simulink model "gait_testing"  (R2024a)
settings: Solver=ode23t  StartTime=0.0  StopTime=8  RelTol=1e-3  AbsTol=1e-3  EnableMultiTasking=on
model workspace (MAT data in the model file):
  A = 0.4
  Length_torso : Simulink.Parameter (value not decoded)
  Lower_limbs : Simulink.Parameter (value not decoded)
  Upper_limbs : Simulink.Parameter (value not decoded)
  Width_torso : Simulink.Parameter (value not decoded)
  f = 1.5
  r_foot : Simulink.Parameter (value not decoded)
  t_leg : Simulink.Parameter (value not decoded)
symbols that are objects in the model workspace (value not decoded): Length_torso, Lower_limbs, t_leg, Upper_limbs, Width_torso
undefined symbols (not defined in the file): P0x, P0z, P1x, P1z, P2x, P2z, X, Y, Z
libraries: sm_lib x88, functionAngles x16, functionAnglesSide x16, nesl_utility x15
(part 9 of 10)

== system gait_testing/Gait Selector/Walk Left Gait - Bezier Curves/Plane Movement/Subsystem1 ==
  X(t) : Inport
  Y(t) : Inport  Port=2
  Add : Sum  Inputs=+--+
  Add1 : Sum
  Add2 : Sum
  Asin : Trigonometry  Operator=asin
  Asin1 : Trigonometry  Operator=asin
  Cos : Trigonometry  Operator=acos
  Divide : Product  Inputs=*/
  Divide1 : Product  Inputs=*/
  Gain : Gain  Gain=1/(2*Upper_limbs*Lower_limbs)
  Gain1 : Gain  Gain=Lower_limbs
  Length lower Limb : Constant  Value=Lower_limbs
  Length upper Limb : Constant  Value=Upper_limbs
  Sin : Trigonometry
  Square{,1..3} (4 alike) : Math  Operator=square
  Square Root : Sqrt
  Theta1(X,Y) : Outport
  Theta2(X,Y) : Outport  Port=2
  wires:
  X(t)/1 -> Divide/1, Square/1
  Y(t)/1 -> Square1/1
  Square/1 -> Add1/1, Add/1
  Length upper Limb/1 -> Square2/1
  Length lower Limb/1 -> Square3/1
  Square2/1 -> Add/2
  Square3/1 -> Add/3
  Square1/1 -> Add1/2, Add/4
  Add/1 -> Gain/1
  Gain/1 -> Cos/1
  Cos/1 -> Theta2(X,Y)/1, Sin/1
  Asin/1 -> Add2/1
  Sin/1 -> Gain1/1
  Add1/1 -> Square Root/1
  Gain1/1 -> Divide1/1
  Square Root/1 -> Divide/2, Divide1/2
  Divide1/1 -> Asin1/1
  Asin1/1 -> Add2/2
  Add2/1 -> Theta1(X,Y)/1
  Divide/1 -> Asin/1

== system gait_testing/Gait Selector/Walk Left Gait - Bezier Curves/Plane Movement1/Subsystem1 ==
  X(t) : Inport
  Y(t) : Inport  Port=2
  Add : Sum  Inputs=+--+
  Add1 : Sum
  Add2 : Sum
  Asin : Trigonometry  Operator=asin
  Asin1 : Trigonometry  Operator=asin
  Cos : Trigonometry  Operator=acos
  Divide : Product  Inputs=*/
  Divide1 : Product  Inputs=*/
  Gain : Gain  Gain=1/(2*Upper_limbs*Lower_limbs)
  Gain1 : Gain  Gain=Lower_limbs
  Length lower Limb : Constant  Value=Lower_limbs
  Length upper Limb : Constant  Value=Upper_limbs
  Sin : Trigonometry
  Square{,1..3} (4 alike) : Math  Operator=square
  Square Root : Sqrt
  Theta1(X,Y) : Outport
  Theta2(X,Y) : Outport  Port=2
  wires:
  X(t)/1 -> Divide/1, Square/1
  Y(t)/1 -> Square1/1
  Square/1 -> Add1/1, Add/1
  Length upper Limb/1 -> Square2/1
  Length lower Limb/1 -> Square3/1
  Square2/1 -> Add/2
  Square3/1 -> Add/3
  Square1/1 -> Add1/2, Add/4
  Add/1 -> Gain/1
  Gain/1 -> Cos/1
  Cos/1 -> Theta2(X,Y)/1, Sin/1
  Asin/1 -> Add2/1
  Sin/1 -> Gain1/1
  Add1/1 -> Square Root/1
  Gain1/1 -> Divide1/1
  Square Root/1 -> Divide/2, Divide1/2
  Divide1/1 -> Asin1/1
  Asin1/1 -> Add2/2
  Add2/1 -> Theta1(X,Y)/1
  Divide/1 -> Asin/1

== system gait_testing/Gait Selector/Walk Left Gait - Bezier Curves/Plane Movement2/Subsystem1 ==
  X(t) : Inport
  Y(t) : Inport  Port=2
  Add : Sum  Inputs=+--+
  Add1 : Sum
  Add2 : Sum
  Asin : Trigonometry  Operator=asin
  Asin1 : Trigonometry  Operator=asin
  Cos : Trigonometry  Operator=acos
  Divide : Product  Inputs=*/
  Divide1 : Product  Inputs=*/
  Gain : Gain  Gain=1/(2*Upper_limbs*Lower_limbs)
  Gain1 : Gain  Gain=Lower_limbs
  Length lower Limb : Constant  Value=Lower_limbs
  Length upper Limb : Constant  Value=Upper_limbs
  Sin : Trigonometry
  Square{,1..3} (4 alike) : Math  Operator=square
  Square Root : Sqrt
  Theta1(X,Y) : Outport
  Theta2(X,Y) : Outport  Port=2
  wires:
  Divide/1 -> Asin/1
  Add2/1 -> Theta1(X,Y)/1
  Asin1/1 -> Add2/2
  Divide1/1 -> Asin1/1
  Square Root/1 -> Divide1/2, Divide/2
  Gain1/1 -> Divide1/1
  Add1/1 -> Square Root/1
  Sin/1 -> Gain1/1
  Asin/1 -> Add2/1
  Cos/1 -> Sin/1, Theta2(X,Y)/1
  Gain/1 -> Cos/1
  Add/1 -> Gain/1
  Square1/1 -> Add/4, Add1/2
  Square3/1 -> Add/3
  Square2/1 -> Add/2
  Length lower Limb/1 -> Square3/1
  Length upper Limb/1 -> Square2/1
  Square/1 -> Add/1, Add1/1
  Y(t)/1 -> Square1/1
  X(t)/1 -> Square/1, Divide/1

== system gait_testing/Gait Selector/Walk Left Gait - Bezier Curves/Plane Movement3/Subsystem1 ==
  X(t) : Inport
  Y(t) : Inport  Port=2
  Add : Sum  Inputs=+--+
  Add1 : Sum
  Add2 : Sum
  Asin : Trigonometry  Operator=asin
  Asin1 : Trigonometry  Operator=asin
  Cos : Trigonometry  Operator=acos
  Divide : Product  Inputs=*/
  Divide1 : Product  Inputs=*/
  Gain : Gain  Gain=1/(2*Upper_limbs*Lower_limbs)
  Gain1 : Gain  Gain=Lower_limbs
  Length lower Limb : Constant  Value=Lower_limbs
  Length upper Limb : Constant  Value=Upper_limbs
  Sin : Trigonometry
  Square{,1..3} (4 alike) : Math  Operator=square
  Square Root : Sqrt
  Theta1(X,Y) : Outport
  Theta2(X,Y) : Outport  Port=2
  wires:
  X(t)/1 -> Divide/1, Square/1
  Y(t)/1 -> Square1/1
  Square/1 -> Add1/1, Add/1
  Length upper Limb/1 -> Square2/1
  Length lower Limb/1 -> Square3/1
  Square2/1 -> Add/2
  Square3/1 -> Add/3
  Square1/1 -> Add1/2, Add/4
  Add/1 -> Gain/1
  Gain/1 -> Cos/1
  Cos/1 -> Theta2(X,Y)/1, Sin/1
  Asin/1 -> Add2/1
  Sin/1 -> Gain1/1
  Add1/1 -> Square Root/1
  Gain1/1 -> Divide1/1
  Square Root/1 -> Divide/2, Divide1/2
  Divide1/1 -> Asin1/1
  Asin1/1 -> Add2/2
  Add2/1 -> Theta1(X,Y)/1
  Divide/1 -> Asin/1

== system gait_testing/Gait Selector/Walk Left Gait - Bezier Curves/Plane Movement4/Subsystem1 ==
  X(t) : Inport
  Y(t) : Inport  Port=2
  Add : Sum  Inputs=+--+
  Add1 : Sum
  Add2 : Sum
  Asin : Trigonometry  Operator=asin
  Asin1 : Trigonometry  Operator=asin
  Cos : Trigonometry  Operator=acos
  Divide : Product  Inputs=*/
  Divide1 : Product  Inputs=*/
  Gain : Gain  Gain=1/(2*Upper_limbs*Lower_limbs)
  Gain1 : Gain  Gain=Lower_limbs
  Length lower Limb : Constant  Value=Lower_limbs
  Length upper Limb : Constant  Value=Upper_limbs
  Sin : Trigonometry
  Square{,1..3} (4 alike) : Math  Operator=square
  Square Root : Sqrt
  Theta1(X,Y) : Outport
  Theta2(X,Y) : Outport  Port=2
  wires:
  Divide/1 -> Asin/1
  Add2/1 -> Theta1(X,Y)/1
  Asin1/1 -> Add2/2
  Divide1/1 -> Asin1/1
  Square Root/1 -> Divide1/2, Divide/2
  Gain1/1 -> Divide1/1
  Add1/1 -> Square Root/1
  Sin/1 -> Gain1/1
  Asin/1 -> Add2/1
  Cos/1 -> Sin/1, Theta2(X,Y)/1
  Gain/1 -> Cos/1
  Add/1 -> Gain/1
  Square1/1 -> Add/4, Add1/2
  Square3/1 -> Add/3
  Square2/1 -> Add/2
  Length lower Limb/1 -> Square3/1
  Length upper Limb/1 -> Square2/1
  Square/1 -> Add/1, Add1/1
  Y(t)/1 -> Square1/1
  X(t)/1 -> Square/1, Divide/1

== system gait_testing/Gait Selector/Walk Left Gait - Bezier Curves/Sin-Movement/Subsystem1 ==
  X(t) : Inport
  Y(t) : Inport  Port=2
  Add : Sum  Inputs=+--+
  Add1 : Sum
  Add2 : Sum
  Asin : Trigonometry  Operator=asin
  Asin1 : Trigonometry  Operator=asin
  Cos : Trigonometry  Operator=acos
  Divide : Product  Inputs=*/
  Divide1 : Product  Inputs=*/
  Gain : Gain  Gain=1/(2*Upper_limbs*Lower_limbs)
  Gain1 : Gain  Gain=Lower_limbs
  Length lower Limb : Constant  Value=Lower_limbs
  Length upper Limb : Constant  Value=Upper_limbs
  Sin : Trigonometry
  Square{,1..3} (4 alike) : Math  Operator=square
  Square Root : Sqrt
  Theta1(X,Y) : Outport
  Theta2(X,Y) : Outport  Port=2
  wires:
  X(t)/1 -> Divide/1, Square/1
  Y(t)/1 -> Square1/1
  Square/1 -> Add1/1, Add/1
  Length upper Limb/1 -> Square2/1
  Length lower Limb/1 -> Square3/1
  Square2/1 -> Add/2
  Square3/1 -> Add/3
  Square1/1 -> Add1/2, Add/4
  Add/1 -> Gain/1
  Gain/1 -> Cos/1
  Cos/1 -> Theta2(X,Y)/1, Sin/1
  Asin/1 -> Add2/1
  Sin/1 -> Gain1/1
  Add1/1 -> Square Root/1
  Gain1/1 -> Divide1/1
  Square Root/1 -> Divide/2, Divide1/2
  Divide1/1 -> Asin1/1
  Asin1/1 -> Add2/2
  Add2/1 -> Theta1(X,Y)/1
  Divide/1 -> Asin/1

== system gait_testing/Gait Selector/Walk Left Gait - Bezier Curves/Stop when change/Triggered Subsystem ==
  t : Inport
  Action Port : ActionPort  InitializeStates=reset  ActionPortLabel=case [ 1 ]:
  MATLAB Function : MATLAB Function  TreatAsAtomicUnit=on
  Change Time : Outport
  wires:
  MATLAB Function/1(activationTime) -> Change Time/1
  t/1 -> MATLAB Function/1(u)

== system gait_testing/Gait Selector/Walk Left Gait - Bezier Curves/delay and stop when change/Triggered Subsystem ==
  t : Inport
  Action Port : ActionPort  InitializeStates=reset  ActionPortLabel=case [ 1 ]:
  MATLAB Function : MATLAB Function  TreatAsAtomicUnit=on
  Change Time : Outport
  wires:
  MATLAB Function/1(activationTime) -> Change Time/1
  t/1 -> MATLAB Function/1(u)

== system gait_testing/Gait Selector/Walk Left Gait - Bezier Curves/delay and stop when change1/Triggered Subsystem ==
  t : Inport
  Action Port : ActionPort  InitializeStates=reset  ActionPortLabel=case [ 1 ]:
  MATLAB Function : MATLAB Function  TreatAsAtomicUnit=on
  Change Time : Outport
  wires:
  MATLAB Function/1(activationTime) -> Change Time/1
  t/1 -> MATLAB Function/1(u)

== system gait_testing/Gait Selector/Walk Left Gait - Bezier Curves/delay and stop when change2/Triggered Subsystem ==
  t : Inport
  Action Port : ActionPort  InitializeStates=reset  ActionPortLabel=case [ 1 ]:
  MATLAB Function : MATLAB Function  TreatAsAtomicUnit=on
  Change Time : Outport
  wires:
  MATLAB Function/1(activationTime) -> Change Time/1
  t/1 -> MATLAB Function/1(u)

== system gait_testing/Gait Selector/Walk Right Gait - Bezier Curves/Plane Movement/Subsystem1 ==
  X(t) : Inport
  Y(t) : Inport  Port=2
  Add : Sum  Inputs=+--+
  Add1 : Sum
  Add2 : Sum
  Asin : Trigonometry  Operator=asin
  Asin1 : Trigonometry  Operator=asin
  Cos : Trigonometry  Operator=acos
  Divide : Product  Inputs=*/
  Divide1 : Product  Inputs=*/
  Gain : Gain  Gain=1/(2*Upper_limbs*Lower_limbs)
  Gain1 : Gain  Gain=Lower_limbs
  Length lower Limb : Constant  Value=Lower_limbs
  Length upper Limb : Constant  Value=Upper_limbs
  Sin : Trigonometry
  Square{,1..3} (4 alike) : Math  Operator=square
  Square Root : Sqrt
  Theta1(X,Y) : Outport
  Theta2(X,Y) : Outport  Port=2
  wires:
  Divide/1 -> Asin/1
  Add2/1 -> Theta1(X,Y)/1
  Asin1/1 -> Add2/2
  Divide1/1 -> Asin1/1
  Square Root/1 -> Divide1/2, Divide/2
  Gain1/1 -> Divide1/1
  Add1/1 -> Square Root/1
  Sin/1 -> Gain1/1
  Asin/1 -> Add2/1
  Cos/1 -> Sin/1, Theta2(X,Y)/1
  Gain/1 -> Cos/1
  Add/1 -> Gain/1
  Square1/1 -> Add/4, Add1/2
  Square3/1 -> Add/3
  Square2/1 -> Add/2
  Length lower Limb/1 -> Square3/1
  Length upper Limb/1 -> Square2/1
  Square/1 -> Add/1, Add1/1
  Y(t)/1 -> Square1/1
  X(t)/1 -> Square/1, Divide/1

== system gait_testing/Gait Selector/Walk Right Gait - Bezier Curves/Plane Movement1/Subsystem1 ==
  X(t) : Inport
  Y(t) : Inport  Port=2
  Add : Sum  Inputs=+--+
  Add1 : Sum
  Add2 : Sum
  Asin : Trigonometry  Operator=asin
  Asin1 : Trigonometry  Operator=asin
  Cos : Trigonometry  Operator=acos
  Divide : Product  Inputs=*/
  Divide1 : Product  Inputs=*/
  Gain : Gain  Gain=1/(2*Upper_limbs*Lower_limbs)
  Gain1 : Gain  Gain=Lower_limbs
  Length lower Limb : Constant  Value=Lower_limbs
  Length upper Limb : Constant  Value=Upper_limbs
  Sin : Trigonometry
  Square{,1..3} (4 alike) : Math  Operator=square
  Square Root : Sqrt
  Theta1(X,Y) : Outport
  Theta2(X,Y) : Outport  Port=2
  wires:
  Divide/1 -> Asin/1
  Add2/1 -> Theta1(X,Y)/1
  Asin1/1 -> Add2/2
  Divide1/1 -> Asin1/1
  Square Root/1 -> Divide1/2, Divide/2
  Gain1/1 -> Divide1/1
  Add1/1 -> Square Root/1
  Sin/1 -> Gain1/1
  Asin/1 -> Add2/1
  Cos/1 -> Sin/1, Theta2(X,Y)/1
  Gain/1 -> Cos/1
  Add/1 -> Gain/1
  Square1/1 -> Add/4, Add1/2
  Square3/1 -> Add/3
  Square2/1 -> Add/2
  Length lower Limb/1 -> Square3/1
  Length upper Limb/1 -> Square2/1
  Square/1 -> Add/1, Add1/1
  Y(t)/1 -> Square1/1
  X(t)/1 -> Square/1, Divide/1

== system gait_testing/Gait Selector/Walk Right Gait - Bezier Curves/Plane Movement2/Subsystem1 ==
  X(t) : Inport
  Y(t) : Inport  Port=2
  Add : Sum  Inputs=+--+
  Add1 : Sum
  Add2 : Sum
  Asin : Trigonometry  Operator=asin
  Asin1 : Trigonometry  Operator=asin
  Cos : Trigonometry  Operator=acos
  Divide : Product  Inputs=*/
  Divide1 : Product  Inputs=*/
  Gain : Gain  Gain=1/(2*Upper_limbs*Lower_limbs)
  Gain1 : Gain  Gain=Lower_limbs
  Length lower Limb : Constant  Value=Lower_limbs
  Length upper Limb : Constant  Value=Upper_limbs
  Sin : Trigonometry
  Square{,1..3} (4 alike) : Math  Operator=square
  Square Root : Sqrt
  Theta1(X,Y) : Outport
  Theta2(X,Y) : Outport  Port=2
  wires:
  X(t)/1 -> Divide/1, Square/1
  Y(t)/1 -> Square1/1
  Square/1 -> Add1/1, Add/1
  Length upper Limb/1 -> Square2/1
  Length lower Limb/1 -> Square3/1
  Square2/1 -> Add/2
  Square3/1 -> Add/3
  Square1/1 -> Add1/2, Add/4
  Add/1 -> Gain/1
  Gain/1 -> Cos/1
  Cos/1 -> Theta2(X,Y)/1, Sin/1
  Asin/1 -> Add2/1
  Sin/1 -> Gain1/1
  Add1/1 -> Square Root/1
  Gain1/1 -> Divide1/1
  Square Root/1 -> Divide/2, Divide1/2
  Divide1/1 -> Asin1/1
  Asin1/1 -> Add2/2
  Add2/1 -> Theta1(X,Y)/1
  Divide/1 -> Asin/1

== system gait_testing/Gait Selector/Walk Right Gait - Bezier Curves/Plane Movement3/Subsystem1 ==
  X(t) : Inport
  Y(t) : Inport  Port=2
  Add : Sum  Inputs=+--+
  Add1 : Sum
  Add2 : Sum
  Asin : Trigonometry  Operator=asin
  Asin1 : Trigonometry  Operator=asin
  Cos : Trigonometry  Operator=acos
  Divide : Product  Inputs=*/
  Divide1 : Product  Inputs=*/
  Gain : Gain  Gain=1/(2*Upper_limbs*Lower_limbs)
  Gain1 : Gain  Gain=Lower_limbs
  Length lower Limb : Constant  Value=Lower_limbs
  Length upper Limb : Constant  Value=Upper_limbs
  Sin : Trigonometry
  Square{,1..3} (4 alike) : Math  Operator=square
  Square Root : Sqrt
  Theta1(X,Y) : Outport
  Theta2(X,Y) : Outport  Port=2
  wires:
  Divide/1 -> Asin/1
  Add2/1 -> Theta1(X,Y)/1
  Asin1/1 -> Add2/2
  Divide1/1 -> Asin1/1
  Square Root/1 -> Divide1/2, Divide/2
  Gain1/1 -> Divide1/1
  Add1/1 -> Square Root/1
  Sin/1 -> Gain1/1
  Asin/1 -> Add2/1
  Cos/1 -> Sin/1, Theta2(X,Y)/1
  Gain/1 -> Cos/1
  Add/1 -> Gain/1
  Square1/1 -> Add/4, Add1/2
  Square3/1 -> Add/3
  Square2/1 -> Add/2
  Length lower Limb/1 -> Square3/1
  Length upper Limb/1 -> Square2/1
  Square/1 -> Add/1, Add1/1
  Y(t)/1 -> Square1/1
  X(t)/1 -> Square/1, Divide/1

== system gait_testing/Gait Selector/Walk Right Gait - Bezier Curves/Plane Movement4/Subsystem1 ==
  X(t) : Inport
  Y(t) : Inport  Port=2
  Add : Sum  Inputs=+--+
  Add1 : Sum
  Add2 : Sum
  Asin : Trigonometry  Operator=asin
  Asin1 : Trigonometry  Operator=asin
  Cos : Trigonometry  Operator=acos
  Divide : Product  Inputs=*/
  Divide1 : Product  Inputs=*/
  Gain : Gain  Gain=1/(2*Upper_limbs*Lower_limbs)
  Gain1 : Gain  Gain=Lower_limbs
  Length lower Limb : Constant  Value=Lower_limbs
  Length upper Limb : Constant  Value=Upper_limbs
  Sin : Trigonometry
  Square{,1..3} (4 alike) : Math  Operator=square
  Square Root : Sqrt
  Theta1(X,Y) : Outport
  Theta2(X,Y) : Outport  Port=2
  wires:
  X(t)/1 -> Divide/1, Square/1
  Y(t)/1 -> Square1/1
  Square/1 -> Add1/1, Add/1
  Length upper Limb/1 -> Square2/1
  Length lower Limb/1 -> Square3/1
  Square2/1 -> Add/2
  Square3/1 -> Add/3
  Square1/1 -> Add1/2, Add/4
  Add/1 -> Gain/1
  Gain/1 -> Cos/1
  Cos/1 -> Theta2(X,Y)/1, Sin/1
  Asin/1 -> Add2/1
  Sin/1 -> Gain1/1
  Add1/1 -> Square Root/1
  Gain1/1 -> Divide1/1
  Square Root/1 -> Divide/2, Divide1/2
  Divide1/1 -> Asin1/1
  Asin1/1 -> Add2/2
  Add2/1 -> Theta1(X,Y)/1
  Divide/1 -> Asin/1

== system gait_testing/Gait Selector/Walk Right Gait - Bezier Curves/Sin-Movement/Subsystem1 ==
  X(t) : Inport
  Y(t) : Inport  Port=2
  Add : Sum  Inputs=+--+
  Add1 : Sum
  Add2 : Sum
  Asin : Trigonometry  Operator=asin
  Asin1 : Trigonometry  Operator=asin
  Cos : Trigonometry  Operator=acos
  Divide : Product  Inputs=*/
  Divide1 : Product  Inputs=*/
  Gain : Gain  Gain=1/(2*Upper_limbs*Lower_limbs)
  Gain1 : Gain  Gain=Lower_limbs
  Length lower Limb : Constant  Value=Lower_limbs
  Length upper Limb : Constant  Value=Upper_limbs
  Sin : Trigonometry
  Square{,1..3} (4 alike) : Math  Operator=square
  Square Root : Sqrt
  Theta1(X,Y) : Outport
  Theta2(X,Y) : Outport  Port=2
  wires:
  Divide/1 -> Asin/1
  Add2/1 -> Theta1(X,Y)/1
  Asin1/1 -> Add2/2
  Divide1/1 -> Asin1/1
  Square Root/1 -> Divide1/2, Divide/2
  Gain1/1 -> Divide1/1
  Add1/1 -> Square Root/1
  Sin/1 -> Gain1/1
  Asin/1 -> Add2/1
  Cos/1 -> Sin/1, Theta2(X,Y)/1
  Gain/1 -> Cos/1
  Add/1 -> Gain/1
  Square1/1 -> Add/4, Add1/2
  Square3/1 -> Add/3
  Square2/1 -> Add/2
  Length lower Limb/1 -> Square3/1
  Length upper Limb/1 -> Square2/1
  Square/1 -> Add/1, Add1/1
  Y(t)/1 -> Square1/1
  X(t)/1 -> Square/1, Divide/1

== system gait_testing/Gait Selector/Walk Right Gait - Bezier Curves/Stop when change/Triggered Subsystem ==
  t : Inport
  Action Port : ActionPort  InitializeStates=reset  ActionPortLabel=case [ 1 ]:
  MATLAB Function : MATLAB Function  TreatAsAtomicUnit=on
  Change Time : Outport
  wires:
  MATLAB Function/1(activationTime) -> Change Time/1
  t/1 -> MATLAB Function/1(u)

== system gait_testing/Gait Selector/Walk Right Gait - Bezier Curves/delay and stop when change/Triggered Subsystem ==
  t : Inport
  Action Port : ActionPort  InitializeStates=reset  ActionPortLabel=case [ 1 ]:
  MATLAB Function : MATLAB Function  TreatAsAtomicUnit=on
  Change Time : Outport
  wires:
  MATLAB Function/1(activationTime) -> Change Time/1
  t/1 -> MATLAB Function/1(u)

== system gait_testing/Gait Selector/Walk Right Gait - Bezier Curves/delay and stop when change1/Triggered Subsystem ==
  t : Inport
  Action Port : ActionPort  InitializeStates=reset  ActionPortLabel=case [ 1 ]:
  MATLAB Function : MATLAB Function  TreatAsAtomicUnit=on
  Change Time : Outport
  wires:
  MATLAB Function/1(activationTime) -> Change Time/1
  t/1 -> MATLAB Function/1(u)

== system gait_testing/Gait Selector/Walk Right Gait - Bezier Curves/delay and stop when change2/Triggered Subsystem ==
  t : Inport
  Action Port : ActionPort  InitializeStates=reset  ActionPortLabel=case [ 1 ]:
  MATLAB Function : MATLAB Function  TreatAsAtomicUnit=on
  Change Time : Outport
  wires:
  MATLAB Function/1(activationTime) -> Change Time/1
  t/1 -> MATLAB Function/1(u)

== matlab function gait_testing/Gait Selector/Walk Gait - Bezier Curves/delay and stop when change/Triggered Subsystem/MATLAB Function ==
  data: u input; activationTime output
function activationTime = getActivationTime(u)
    persistent t_start
    if isempty(t_start)
        t_start = u;
    end
    activationTime = t_start;
end

== matlab function gait_testing/Gait Selector/Walk Gait - Bezier Curves/delay and stop when change1/Triggered Subsystem/MATLAB Function ==
  data: u input; activationTime output
function activationTime = getActivationTime(u)
    persistent t_start
    if isempty(t_start)
        t_start = u;
    end
    activationTime = t_start;
end

== matlab function gait_testing/Gait Selector/Walk Gait - Bezier Curves/delay and stop when change2/Triggered Subsystem/MATLAB Function ==
  data: u input; activationTime output
function activationTime = getActivationTime(u)
    persistent t_start
    if isempty(t_start)
        t_start = u;
    end
    activationTime = t_start;
end

== matlab function gait_testing/Gait Selector/MATLAB Function ==
  data: c_old input; c_new input; t input; C_out output; t_change input; tdur_old input; tdur_new input; tdur_out output
function [C_out, tdur_out]= control_change(c_old, c_new, t, t_change, tdur_old, tdur_new)

time_since_change = t-t_change;
if c_old == 0 || t < tdur_old
    C_out = c_new;
    tdur_out = tdur_new;

else
    if time_since_change < tdur_old
        C_out = c_old;
        tdur_out = tdur_old;
    else
        if time_since_change < (tdur_old+0.05)
            C_out = 0;
            tdur_out = 0.05;
        else
            C_out = c_new;
            tdur_out = tdur_new;
        end
    end

end
end

== matlab function gait_testing/Gait Selector/Trot Gait - Bezier Curves/Stop when change/Triggered Subsystem/MATLAB Function ==
  data: u input; activationTime output
function activationTime = getActivationTime(u)
    persistent t_start
    if isempty(t_start)
        t_start = u;
    end
    activationTime = t_start;
end

== matlab function gait_testing/Gait Selector/Trot Gait - Bezier Curves/delay and stop when change/Triggered Subsystem/MATLAB Function ==
  data: u input; activationTime output
function activationTime = getActivationTime(u)
    persistent t_start
    if isempty(t_start)
        t_start = u;
    end
    activationTime = t_start;
end

== matlab function gait_testing/Gait Selector/Trot Gait - Bezier Curves/delay and stop when change1/Triggered Subsystem/MATLAB Function ==
  data: u input; activationTime output
function activationTime = getActivationTime(u)
    persistent t_start
    if isempty(t_start)
        t_start = u;
    end
    activationTime = t_start;
end

== matlab function gait_testing/Gait Selector/Trot Gait - Bezier Curves/delay and stop when change2/Triggered Subsystem/MATLAB Function ==
  data: u input; activationTime output
function activationTime = getActivationTime(u)
    persistent t_start
    if isempty(t_start)
        t_start = u;
    end
    activationTime = t_start;
end

== matlab function gait_testing/Gait Selector/Walk Back Gait - Bezier Curves/Stop when change/Triggered Subsystem/MATLAB Function ==
  data: u input; activationTime output
function activationTime = getActivationTime(u)
    persistent t_start
    if isempty(t_start)
        t_start = u;
    end
    activationTime = t_start;
end

== matlab function gait_testing/Gait Selector/Walk Left Gait - Bezier Curves/Plane Movement/MATLAB Function2 ==
  data: x output; t input; Tdur input; y output; P0x input; P0z input; P1x input; P1z input; P2x input; P2z input; P3x input; P3z input
function [x, y] = bez_plane_TrajV2(t,Tdur,P0x,P0z,P1x,P1z,P2x,P2z,P3x,P3z)
t_swing = Tdur/4;
t_support = Tdur*3/4;

P0 = [P0x, P0z];
P1 = [P1x, P1z];
P2 = [P2x, P2z];
P3 = [P3x, P3z];
if t<=t_swing
    Sw = P0*((1-(t/t_swing))^3) + 3*P1*(t/t_swing)*((1-(t/t_swing))^2) + 3*P2*((t/t_swing)^2)*(1-(t/t_swing)) + P3*((t/t_swing)^3);
    
    x = -1*Sw(1);
    y = Sw(2);
else
    x = -1*(P3(1)+(P0(1)-P3(1))/t_support*(t-t_swing));
    y = P0(2);
end
end

== matlab function gait_testing/Gait Selector/Walk Back Gait - Bezier Curves/delay and stop when change/Triggered Subsystem/MATLAB Function ==
  data: u input; activationTime output
function activationTime = getActivationTime(u)
    persistent t_start
    if isempty(t_start)
        t_start = u;
    end
    activationTime = t_start;
end

== matlab function gait_testing/Gait Selector/Walk Back Gait - Bezier Curves/delay and stop when change1/Triggered Subsystem/MATLAB Function ==
  data: u input; activationTime output
function activationTime = getActivationTime(u)
    persistent t_start
    if isempty(t_start)
        t_start = u;
    end
    activationTime = t_start;
end

== matlab function gait_testing/Gait Selector/Walk Back Gait - Bezier Curves/delay and stop when change2/Triggered Subsystem/MATLAB Function ==
  data: u input; activationTime output
function activationTime = getActivationTime(u)
    persistent t_start
    if isempty(t_start)
        t_start = u;
    end
    activationTime = t_start;
end

== matlab function gait_testing/Gait Selector/Walk Left Gait - Bezier Curves/Stop when change/Triggered Subsystem/MATLAB Function ==
  data: u input; activationTime output
function activationTime = getActivationTime(u)
    persistent t_start
    if isempty(t_start)
        t_start = u;
    end
    activationTime = t_start;
end

== matlab function gait_testing/Gait Selector/Walk Left Gait - Bezier Curves/delay and stop when change/Triggered Subsystem/MATLAB Function ==
  data: u input; activationTime output
function activationTime = getActivationTime(u)
    persistent t_start
    if isempty(t_start)
        t_start = u;
    end
    activationTime = t_start;
end

== matlab function gait_testing/Gait Selector/Walk Left Gait - Bezier Curves/delay and stop when change1/Triggered Subsystem/MATLAB Function ==
  data: u input; activationTime output
function activationTime = getActivationTime(u)
    persistent t_start
    if isempty(t_start)
        t_start = u;
    end
    activationTime = t_start;
end

== matlab function gait_testing/Gait Selector/Walk Left Gait - Bezier Curves/delay and stop when change2/Triggered Subsystem/MATLAB Function ==
  data: u input; activationTime output
function activationTime = getActivationTime(u)
    persistent t_start
    if isempty(t_start)
        t_start = u;
    end
    activationTime = t_start;
end

== matlab function gait_testing/Gait Selector/Walk Right Gait - Bezier Curves/Stop when change/Triggered Subsystem/MATLAB Function ==
  data: u input; activationTime output
function activationTime = getActivationTime(u)
    persistent t_start
    if isempty(t_start)
        t_start = u;
    end
    activationTime = t_start;
end

== matlab function gait_testing/Gait Selector/Walk Right Gait - Bezier Curves/delay and stop when change/Triggered Subsystem/MATLAB Function ==
  data: u input; activationTime output
function activationTime = getActivationTime(u)
    persistent t_start
    if isempty(t_start)
        t_start = u;
    end
    activationTime = t_start;
end

== matlab function gait_testing/Gait Selector/Walk Right Gait - Bezier Curves/delay and stop when change1/Triggered Subsystem/MATLAB Function ==
  data: u input; activationTime output
function activationTime = getActivationTime(u)
    persistent t_start
    if isempty(t_start)
        t_start = u;
    end
    activationTime = t_start;
end

== matlab function gait_testing/Gait Selector/Walk Right Gait - Bezier Curves/delay and stop when change2/Triggered Subsystem/MATLAB Function ==
  data: u input; activationTime output
function activationTime = getActivationTime(u)
    persistent t_start
    if isempty(t_start)
        t_start = u;
    end
    activationTime = t_start;
end

== matlab function gait_testing/Gait Selector/Turn Left Gait - Bezier Curves/Stop when change/Triggered Subsystem/MATLAB Function ==
  data: u input; activationTime output
function activationTime = getActivationTime(u)
    persistent t_start
    if isempty(t_start)
        t_start = u;
    end
    activationTime = t_start;
end

== matlab function gait_testing/Gait Selector/Turn Left Gait - Bezier Curves/delay and stop when change/Triggered Subsystem/MATLAB Function ==
  data: u input; activationTime output
function activationTime = getActivationTime(u)
    persistent t_start
    if isempty(t_start)
        t_start = u;
    end
    activationTime = t_start;
end

== matlab function gait_testing/Gait Selector/Turn Left Gait - Bezier Curves/delay and stop when change1/Triggered Subsystem/MATLAB Function ==
  data: u input; activationTime output
function activationTime = getActivationTime(u)
    persistent t_start
    if isempty(t_start)
        t_start = u;
    end
    activationTime = t_start;
end

== matlab function gait_testing/Gait Selector/Turn Left Gait - Bezier Curves/delay and stop when change2/Triggered Subsystem/MATLAB Function ==
  data: u input; activationTime output
function activationTime = getActivationTime(u)
    persistent t_start
    if isempty(t_start)
        t_start = u;
    end
    activationTime = t_start;
end

== matlab function gait_testing/Gait Selector/Turn Right Gait - Bezier Curves/Stop when change/Triggered Subsystem/MATLAB Function ==
  data: u input; activationTime output
function activationTime = getActivationTime(u)
    persistent t_start
    if isempty(t_start)
        t_start = u;
    end
    activationTime = t_start;
end

== matlab function gait_testing/Gait Selector/Turn Right Gait - Bezier Curves/delay and stop when change/Triggered Subsystem/MATLAB Function ==
  data: u input; activationTime output
function activationTime = getActivationTime(u)
    persistent t_start
    if isempty(t_start)
        t_start = u;
    end
    activationTime = t_start;
end

== matlab function gait_testing/Gait Selector/Turn Right Gait - Bezier Curves/delay and stop when change1/Triggered Subsystem/MATLAB Function ==
  data: u input; activationTime output
function activationTime = getActivationTime(u)
    persistent t_start
    if isempty(t_start)
        t_start = u;
    end
    activationTime = t_start;
end

== matlab function gait_testing/Gait Selector/Turn Right Gait - Bezier Curves/delay and stop when change2/Triggered Subsystem/MATLAB Function ==
  data: u input; activationTime output
function activationTime = getActivationTime(u)
    persistent t_start
    if isempty(t_start)
        t_start = u;
    end
    activationTime = t_start;
end

== matlab function gait_testing/Gait Selector/Trot Gait - Bezier Curves/Plane Movement/MATLAB Function1 ==
  data: x input; theta1 output; y input; L1 input; L2 input; theta2 output
function [theta1, theta2] = ang(x,y,L1,L2)
theta2 = acos((x.^2+y.^2-L1.^2-L2.^2) / (2*L1*L2));
beta = asin((L2*sin(theta2))./((x.^2+y.^2).^0.5));
theta1 = asin(x./((x.^2+y.^2).^0.5)) + beta;
end

== matlab function gait_testing/Gait Selector/Trot Gait - Bezier Curves/Plane Movement/MATLAB Function2 ==
  data: x output; t input; Tdur input; y output; P0x input; P0z input; P1x input; P1z input; P2x input; P2z input; P3x input; P3z input
function [x, y] = bez_plane_TrajV2(t,Tdur,P0x,P0z,P1x,P1z,P2x,P2z,P3x,P3z)
t_swing = Tdur/4;
t_support = Tdur*3/4;

P0 = [P0x, P0z];
P1 = [P1x, P1z];
P2 = [P2x, P2z];
P3 = [P3x, P3z];
if t<=t_swing
    Sw = P0*((1-(t/t_swing))^3) + 3*P1*(t/t_swing)*((1-(t/t_swing))^2) + 3*P2*((t/t_swing)^2)*(1-(t/t_swing)) + P3*((t/t_swing)^3);
    
    x = -1*Sw(1);
    y = Sw(2);
else
    x = -1*(P3(1)+(P0(1)-P3(1))/t_support*(t-t_swing));
    y = P0(2);
end
end

== matlab function gait_testing/Gait Selector/Trot Gait - Bezier Curves/Plane Movement4/MATLAB Function2 ==
  data: x output; t input; Tdur input; y output; P0x input; P0z input; P1x input; P1z input; P2x input; P2z input; P3x input; P3z input
function [x, y] = bez_plane_TrajV2(t,Tdur,P0x,P0z,P1x,P1z,P2x,P2z,P3x,P3z)
t_swing = Tdur/4;
t_support = Tdur*3/4;

P0 = [P0x, P0z];
P1 = [P1x, P1z];
P2 = [P2x, P2z];
P3 = [P3x, P3z];
if t<=t_swing
    Sw = P0*((1-(t/t_swing))^3) + 3*P1*(t/t_swing)*((1-(t/t_swing))^2) + 3*P2*((t/t_swing)^2)*(1-(t/t_swing)) + P3*((t/t_swing)^3);
    
    x = -1*Sw(1);
    y = Sw(2);
else
    x = -1*(P3(1)+(P0(1)-P3(1))/t_support*(t-t_swing));
    y = P0(2);
end
end

== matlab function gait_testing/Gait Selector/Walk Left Gait - Bezier Curves/Plane Movement1/MATLAB Function2 ==
  data: x output; t input; Tdur input; y output; P0x input; P0z input; P1x input; P1z input; P2x input; P2z input; P3x input; P3z input
function [x, y] = bez_plane_TrajV2(t,Tdur,P0x,P0z,P1x,P1z,P2x,P2z,P3x,P3z)
t_swing = Tdur/4;
t_support = Tdur*3/4;

P0 = [P0x, P0z];
P1 = [P1x, P1z];
P2 = [P2x, P2z];
P3 = [P3x, P3z];
if t<=t_swing
    Sw = P0*((1-(t/t_swing))^3) + 3*P1*(t/t_swing)*((1-(t/t_swing))^2) + 3*P2*((t/t_swing)^2)*(1-(t/t_swing)) + P3*((t/t_swing)^3);
    
    x = 1*Sw(1);
    y = Sw(2);
else
    x = 1*(P3(1)+(P0(1)-P3(1))/t_support*(t-t_swing));
    y = P0(2);
end
end

== matlab function gait_testing/Gait Selector/Trot Gait - Bezier Curves/Sin-Movement/MATLAB Function1 ==
  data: x input; theta1 output; y input; L1 input; L2 input; theta2 output
function [theta1, theta2] = ang(x,y,L1,L2)
theta2 = acos((x.^2+y.^2-L1.^2-L2.^2) / (2*L1*L2));
beta = asin((L2*sin(theta2))./((x.^2+y.^2).^0.5));
theta1 = asin(x./((x.^2+y.^2).^0.5)) + beta;
end

== matlab function gait_testing/Gait Selector/Walk Left Gait - Bezier Curves/Plane Movement2/MATLAB Function2 ==
  data: x output; t input; Tdur input; y output; P0x input; P0z input; P1x input; P1z input; P2x input; P2z input; P3x input; P3z input
function [x, y] = bez_plane_TrajV2(t,Tdur,P0x,P0z,P1x,P1z,P2x,P2z,P3x,P3z)
t_swing = Tdur/4;
t_support = Tdur*3/4;

P0 = [P0x, P0z];
P1 = [P1x, P1z];
P2 = [P2x, P2z];
P3 = [P3x, P3z];
if t<=t_swing
    Sw = P0*((1-(t/t_swing))^3) + 3*P1*(t/t_swing)*((1-(t/t_swing))^2) + 3*P2*((t/t_swing)^2)*(1-(t/t_swing)) + P3*((t/t_swing)^3);
    
    x = 1*Sw(1);
    y = Sw(2);
else
    x = 1*(P3(1)+(P0(1)-P3(1))/t_support*(t-t_swing));
    y = P0(2);
end
end

== matlab function gait_testing/Gait Selector/Walk Left Gait - Bezier Curves/Plane Movement3/MATLAB Function2 ==
  data: x output; t input; Tdur input; y output; P0x input; P0z input; P1x input; P1z input; P2x input; P2z input; P3x input; P3z input
function [x, y] = bez_plane_TrajV2(t,Tdur,P0x,P0z,P1x,P1z,P2x,P2z,P3x,P3z)
t_swing = Tdur/4;
t_support = Tdur*3/4;

P0 = [P0x, P0z];
P1 = [P1x, P1z];
P2 = [P2x, P2z];
P3 = [P3x, P3z];
if t<=t_swing
    Sw = P0*((1-(t/t_swing))^3) + 3*P1*(t/t_swing)*((1-(t/t_swing))^2) + 3*P2*((t/t_swing)^2)*(1-(t/t_swing)) + P3*((t/t_swing)^3);
    
    x = 1*Sw(1);
    y = Sw(2);
else
    x = 1*(P3(1)+(P0(1)-P3(1))/t_support*(t-t_swing));
    y = P0(2);
end
end

== matlab function gait_testing/Gait Selector/Walk Left Gait - Bezier Curves/Plane Movement4/MATLAB Function2 ==
  data: x output; t input; Tdur input; y output; P0x input; P0z input; P1x input; P1z input; P2x input; P2z input; P3x input; P3z input
function [x, y] = bez_plane_TrajV2(t,Tdur,P0x,P0z,P1x,P1z,P2x,P2z,P3x,P3z)
t_swing = Tdur/4;
t_support = Tdur*3/4;

P0 = [P0x, P0z];
P1 = [P1x, P1z];
P2 = [P2x, P2z];
P3 = [P3x, P3z];
if t<=t_swing
    Sw = P0*((1-(t/t_swing))^3) + 3*P1*(t/t_swing)*((1-(t/t_swing))^2) + 3*P2*((t/t_swing)^2)*(1-(t/t_swing)) + P3*((t/t_swing)^3);
    
    x = 1*Sw(1);
    y = Sw(2);
else
    x = 1*(P3(1)+(P0(1)-P3(1))/t_support*(t-t_swing));
    y = P0(2);
end
end

== matlab function gait_testing/Gait Selector/Walk Left Gait - Bezier Curves/Sin-Movement/MATLAB Function ==
  data: x output; t input; y output; Tdur input; P0x input; P0z input; P1x input; P1z input; P2x input; P2z input; P3x input; P3z input
function [x, y] = bezTrajV2(t, Tdur, P0x,P0z,P1x,P1z,P2x,P2z,P3x,P3z)
t_swing = Tdur/4;
t_support = Tdur*3/4;

P0 = [P0x, P0z];
P1 = [P1x, P1z];
P2 = [P2x, P2z];
P3 = [P3x, P3z];
if t<=t_swing
    Sw = P0*((1-(t/t_swing))^3) + 3*P1*(t/t_swing)*((1-(t/t_swing))^2) + 3*P2*((t/t_swing)^2)*(1-(t/t_swing)) + P3*((t/t_swing)^3);
    
    x = -1*Sw(1);
    y = Sw(2);
else
    x = -1*(P3(1)+(P0(1)-P3(1))/t_support*(t-t_swing));
    y = -0.003*sin((x-P0(1))*pi/(P3(1)-P0(1)))+P0(2);
end
end

== matlab function gait_testing/Gait Selector/Walk Left Gait - Bezier Curves/Sin-Movement/MATLAB Function1 ==
  data: x input; theta1 output; y input; L1 input; L2 input; theta2 output
function [theta1, theta2] = ang(x,y,L1,L2)
theta2 = acos((x.^2+y.^2-L1.^2-L2.^2) / (2*L1*L2));
beta = asin((L2*sin(theta2))./((x.^2+y.^2).^0.5));
theta1 = asin(x./((x.^2+y.^2).^0.5)) + beta;
end

== matlab function gait_testing/Gait Selector/Walk Right Gait - Bezier Curves/Plane Movement/MATLAB Function1 ==
  data: x input; theta1 output; y input; L1 input; L2 input; theta2 output
function [theta1, theta2] = ang(x,y,L1,L2)
theta2 = acos((x.^2+y.^2-L1.^2-L2.^2) / (2*L1*L2));
beta = asin((L2*sin(theta2))./((x.^2+y.^2).^0.5));
theta1 = asin(x./((x.^2+y.^2).^0.5)) + beta;
end

== matlab function gait_testing/Gait Selector/Walk Right Gait - Bezier Curves/Plane Movement/MATLAB Function2 ==
  data: x output; t input; Tdur input; y output; P0x input; P0z input; P1x input; P1z input; P2x input; P2z input; P3x input; P3z input
function [x, y] = bez_plane_TrajV2(t,Tdur,P0x,P0z,P1x,P1z,P2x,P2z,P3x,P3z)
t_swing = Tdur/4;
t_support = Tdur*3/4;

P0 = [P0x, P0z];
P1 = [P1x, P1z];
P2 = [P2x, P2z];
P3 = [P3x, P3z];
if t<=t_swing
    Sw = P0*((1-(t/t_swing))^3) + 3*P1*(t/t_swing)*((1-(t/t_swing))^2) + 3*P2*((t/t_swing)^2)*(1-(t/t_swing)) + P3*((t/t_swing)^3);
    
    x = -1*Sw(1);
    y = Sw(2);
else
    x = -1*(P3(1)+(P0(1)-P3(1))/t_support*(t-t_swing));
    y = P0(2);
end
end

== matlab function gait_testing/Gait Selector/Trot Gait - Bezier Curves/Sin-Movement/MATLAB Function ==
  data: x output; t input; y output; Tdur input; P0x input; P0z input; P1x input; P1z input; P2x input; P2z input; P3x input; P3z input
function [x, y] = bezTrajV2(t, Tdur, P0x,P0z,P1x,P1z,P2x,P2z,P3x,P3z)
t_swing = Tdur/4;
t_support = Tdur*3/4;

P0 = [P0x, P0z];
P1 = [P1x, P1z];
P2 = [P2x, P2z];
P3 = [P3x, P3z];
if t<=t_swing
    Sw = P0*((1-(t/t_swing))^3) + 3*P1*(t/t_swing)*((1-(t/t_swing))^2) + 3*P2*((t/t_swing)^2)*(1-(t/t_swing)) + P3*((t/t_swing)^3);
    
    x = -1*Sw(1);
    y = Sw(2);
else
    x = -1*(P3(1)+(P0(1)-P3(1))/t_support*(t-t_swing));
    y = -0.003*sin((x-P0(1))*pi/(P3(1)-P0(1)))+P0(2);
end
end

== matlab function gait_testing/Gait Selector/Walk Right Gait - Bezier Curves/Plane Movement1/MATLAB Function2 ==
  data: x output; t input; Tdur input; y output; P0x input; P0z input; P1x input; P1z input; P2x input; P2z input; P3x input; P3z input
function [x, y] = bez_plane_TrajV2(t,Tdur,P0x,P0z,P1x,P1z,P2x,P2z,P3x,P3z)
t_swing = Tdur/4;
t_support = Tdur*3/4;

P0 = [P0x, P0z];
P1 = [P1x, P1z];
P2 = [P2x, P2z];
P3 = [P3x, P3z];
if t<=t_swing
    Sw = P0*((1-(t/t_swing))^3) + 3*P1*(t/t_swing)*((1-(t/t_swing))^2) + 3*P2*((t/t_swing)^2)*(1-(t/t_swing)) + P3*((t/t_swing)^3);
    
    x = -1*Sw(1);
    y = Sw(2);
else
    x = -1*(P3(1)+(P0(1)-P3(1))/t_support*(t-t_swing));
    y = P0(2);
end
end

== matlab function gait_testing/Gait Selector/Walk Right Gait - Bezier Curves/Plane Movement2/MATLAB Function2 ==
  data: x output; t input; Tdur input; y output; P0x input; P0z input; P1x input; P1z input; P2x input; P2z input; P3x input; P3z input
function [x, y] = bez_plane_TrajV2(t,Tdur,P0x,P0z,P1x,P1z,P2x,P2z,P3x,P3z)
t_swing = Tdur/4;
t_support = Tdur*3/4;

P0 = [P0x, P0z];
P1 = [P1x, P1z];
P2 = [P2x, P2z];
P3 = [P3x, P3z];
if t<=t_swing
    Sw = P0*((1-(t/t_swing))^3) + 3*P1*(t/t_swing)*((1-(t/t_swing))^2) + 3*P2*((t/t_swing)^2)*(1-(t/t_swing)) + P3*((t/t_swing)^3);
    
    x = -1*Sw(1);
    y = Sw(2);
else
    x = -1*(P3(1)+(P0(1)-P3(1))/t_support*(t-t_swing));
    y = P0(2);
end
end

== matlab function gait_testing/Gait Selector/Walk Right Gait - Bezier Curves/Plane Movement3/MATLAB Function2 ==
  data: x output; t input; Tdur input; y output; P0x input; P0z input; P1x input; P1z input; P2x input; P2z input; P3x input; P3z input
function [x, y] = bez_plane_TrajV2(t,Tdur,P0x,P0z,P1x,P1z,P2x,P2z,P3x,P3z)
t_swing = Tdur/4;
t_support = Tdur*3/4;

P0 = [P0x, P0z];
P1 = [P1x, P1z];
P2 = [P2x, P2z];
P3 = [P3x, P3z];
if t<=t_swing
    Sw = P0*((1-(t/t_swing))^3) + 3*P1*(t/t_swing)*((1-(t/t_swing))^2) + 3*P2*((t/t_swing)^2)*(1-(t/t_swing)) + P3*((t/t_swing)^3);
    
    x = -1*Sw(1);
    y = Sw(2);
else
    x = -1*(P3(1)+(P0(1)-P3(1))/t_support*(t-t_swing));
    y = P0(2);
end
end

== matlab function gait_testing/Gait Selector/Walk Right Gait - Bezier Curves/Plane Movement4/MATLAB Function2 ==
  data: x output; t input; Tdur input; y output; P0x input; P0z input; P1x input; P1z input; P2x input; P2z input; P3x input; P3z input
function [x, y] = bez_plane_TrajV2(t,Tdur,P0x,P0z,P1x,P1z,P2x,P2z,P3x,P3z)
t_swing = Tdur/4;
t_support = Tdur*3/4;

P0 = [P0x, P0z];
P1 = [P1x, P1z];
P2 = [P2x, P2z];
P3 = [P3x, P3z];
if t<=t_swing
    Sw = P0*((1-(t/t_swing))^3) + 3*P1*(t/t_swing)*((1-(t/t_swing))^2) + 3*P2*((t/t_swing)^2)*(1-(t/t_swing)) + P3*((t/t_swing)^3);
    
    x = -1*Sw(1);
    y = Sw(2);
else
    x = -1*(P3(1)+(P0(1)-P3(1))/t_support*(t-t_swing));
    y = P0(2);
end
end

== matlab function gait_testing/Gait Selector/Walk Right Gait - Bezier Curves/Sin-Movement/MATLAB Function ==
  data: x output; t input; y output; Tdur input; P0x input; P0z input; P1x input; P1z input; P2x input; P2z input; P3x input; P3z input
function [x, y] = bezTrajV2(t, Tdur, P0x,P0z,P1x,P1z,P2x,P2z,P3x,P3z)
t_swing = Tdur/4;
t_support = Tdur*3/4;

P0 = [P0x, P0z];
P1 = [P1x, P1z];
P2 = [P2x, P2z];
P3 = [P3x, P3z];
if t<=t_swing
    Sw = P0*((1-(t/t_swing))^3) + 3*P1*(t/t_swing)*((1-(t/t_swing))^2) + 3*P2*((t/t_swing)^2)*(1-(t/t_swing)) + P3*((t/t_swing)^3);
    
    x = -1*Sw(1);
    y = Sw(2);
else
    x = -1*(P3(1)+(P0(1)-P3(1))/t_support*(t-t_swing));
    y = -0.003*sin((x-P0(1))*pi/(P3(1)-P0(1)))+P0(2);
end
end

== matlab function gait_testing/Gait Selector/Walk Right Gait - Bezier Curves/Sin-Movement/MATLAB Function1 ==
  data: x input; theta1 output; y input; L1 input; L2 input; theta2 output
function [theta1, theta2] = ang(x,y,L1,L2)
theta2 = acos((x.^2+y.^2-L1.^2-L2.^2) / (2*L1*L2));
beta = asin((L2*sin(theta2))./((x.^2+y.^2).^0.5));
theta1 = asin(x./((x.^2+y.^2).^0.5)) + beta;
end

== matlab function gait_testing/Gait Selector/Turn Left Gait - Bezier Curves/Plane Movement/MATLAB Function1 ==
  data: x input; theta1 output; y input; L1 input; L2 input; theta2 output
function [theta1, theta2] = ang(x,y,L1,L2)
theta2 = acos((x.^2+y.^2-L1.^2-L2.^2) / (2*L1*L2));
beta = asin((L2*sin(theta2))./((x.^2+y.^2).^0.5));
theta1 = asin(x./((x.^2+y.^2).^0.5)) + beta;
end

== matlab function gait_testing/Gait Selector/Turn Left Gait - Bezier Curves/Plane Movement/MATLAB Function2 ==
  data: x output; t input; Tdur input; y output; P0x input; P0z input; P1x input; P1z input; P2x input; P2z input; P3x input; P3z input
function [x, y] = bez_plane_TrajV2(t,Tdur,P0x,P0z,P1x,P1z,P2x,P2z,P3x,P3z)
t_swing = Tdur/4;
t_support = Tdur*3/4;

P0 = [P0x, P0z];
P1 = [P1x, P1z];
P2 = [P2x, P2z];
P3 = [P3x, P3z];
if t<=t_swing
    Sw = P0*((1-(t/t_swing))^3) + 3*P1*(t/t_swing)*((1-(t/t_swing))^2) + 3*P2*((t/t_swing)^2)*(1-(t/t_swing)) + P3*((t/t_swing)^3);
    
    x = -1*Sw(1);
    y = Sw(2);
else
    x = -1*(P3(1)+(P0(1)-P3(1))/t_support*(t-t_swing));
    y = P0(2);
end
end

== matlab function gait_testing/Gait Selector/Turn Left Gait - Bezier Curves/Plane Movement1/MATLAB Function2 ==
  data: x output; t input; Tdur input; y output; P0x input; P0z input; P1x input; P1z input; P2x input; P2z input; P3x input; P3z input
function [x, y] = bez_plane_TrajV2(t,Tdur,P0x,P0z,P1x,P1z,P2x,P2z,P3x,P3z)
t_swing = Tdur/4;
t_support = Tdur*3/4;

P0 = [P0x, P0z];
P1 = [P1x, P1z];
P2 = [P2x, P2z];
P3 = [P3x, P3z];
if t<=t_swing
    Sw = P0*((1-(t/t_swing))^3) + 3*P1*(t/t_swing)*((1-(t/t_swing))^2) + 3*P2*((t/t_swing)^2)*(1-(t/t_swing)) + P3*((t/t_swing)^3);
    
    x = 1*Sw(1);
    y = Sw(2);
else
    x = 1*(P3(1)+(P0(1)-P3(1))/t_support*(t-t_swing));
    y = P0(2);
end
end

== matlab function gait_testing/Gait Selector/Turn Left Gait - Bezier Curves/Plane Movement2/MATLAB Function2 ==
  data: x output; t input; Tdur input; y output; P0x input; P0z input; P1x input; P1z input; P2x input; P2z input; P3x input; P3z input
function [x, y] = bez_plane_TrajV2(t,Tdur,P0x,P0z,P1x,P1z,P2x,P2z,P3x,P3z)
t_swing = Tdur/4;
t_support = Tdur*3/4;

P0 = [P0x, P0z];
P1 = [P1x, P1z];
P2 = [P2x, P2z];
P3 = [P3x, P3z];
if t<=t_swing
    Sw = P0*((1-(t/t_swing))^3) + 3*P1*(t/t_swing)*((1-(t/t_swing))^2) + 3*P2*((t/t_swing)^2)*(1-(t/t_swing)) + P3*((t/t_swing)^3);
    
    x = -1*Sw(1);
    y = Sw(2);
else
    x = -1*(P3(1)+(P0(1)-P3(1))/t_support*(t-t_swing));
    y = P0(2);
end
end

== matlab function gait_testing/Gait Selector/Trot Gait - Bezier Curves/Plane Movement1/MATLAB Function2 ==
  data: x output; t input; Tdur input; y output; P0x input; P0z input; P1x input; P1z input; P2x input; P2z input; P3x input; P3z input
function [x, y] = bez_plane_TrajV2(t,Tdur,P0x,P0z,P1x,P1z,P2x,P2z,P3x,P3z)
t_swing = Tdur/4;
t_support = Tdur*3/4;

P0 = [P0x, P0z];
P1 = [P1x, P1z];
P2 = [P2x, P2z];
P3 = [P3x, P3z];
if t<=t_swing
    Sw = P0*((1-(t/t_swing))^3) + 3*P1*(t/t_swing)*((1-(t/t_swing))^2) + 3*P2*((t/t_swing)^2)*(1-(t/t_swing)) + P3*((t/t_swing)^3);
    
    x = -1*Sw(1);
    y = Sw(2);
else
    x = -1*(P3(1)+(P0(1)-P3(1))/t_support*(t-t_swing));
    y = P0(2);
end
end

== matlab function gait_testing/Gait Selector/Turn Left Gait - Bezier Curves/Plane Movement3/MATLAB Function2 ==
  data: x output; t input; Tdur input; y output; P0x input; P0z input; P1x input; P1z input; P2x input; P2z input; P3x input; P3z input
function [x, y] = bez_plane_TrajV2(t,Tdur,P0x,P0z,P1x,P1z,P2x,P2z,P3x,P3z)
t_swing = Tdur/4;
t_support = Tdur*3/4;

P0 = [P0x, P0z];
P1 = [P1x, P1z];
P2 = [P2x, P2z];
P3 = [P3x, P3z];
if t<=t_swing
    Sw = P0*((1-(t/t_swing))^3) + 3*P1*(t/t_swing)*((1-(t/t_swing))^2) + 3*P2*((t/t_swing)^2)*(1-(t/t_swing)) + P3*((t/t_swing)^3);
    
    x = -1*Sw(1);
    y = Sw(2);
else
    x = -1*(P3(1)+(P0(1)-P3(1))/t_support*(t-t_swing));
    y = P0(2);
end
end

== matlab function gait_testing/Gait Selector/Turn Left Gait - Bezier Curves/Plane Movement4/MATLAB Function2 ==
  data: x output; t input; Tdur input; y output; P0x input; P0z input; P1x input; P1z input; P2x input; P2z input; P3x input; P3z input
function [x, y] = bez_plane_TrajV2(t,Tdur,P0x,P0z,P1x,P1z,P2x,P2z,P3x,P3z)
t_swing = Tdur/4;
t_support = Tdur*3/4;

P0 = [P0x, P0z];
P1 = [P1x, P1z];
P2 = [P2x, P2z];
P3 = [P3x, P3z];
if t<=t_swing
    Sw = P0*((1-(t/t_swing))^3) + 3*P1*(t/t_swing)*((1-(t/t_swing))^2) + 3*P2*((t/t_swing)^2)*(1-(t/t_swing)) + P3*((t/t_swing)^3);
    
    x = 1*Sw(1);
    y = Sw(2);
else
    x = 1*(P3(1)+(P0(1)-P3(1))/t_support*(t-t_swing));
    y = P0(2);
end
end

== matlab function gait_testing/Gait Selector/Turn Left Gait - Bezier Curves/Sin-Movement/MATLAB Function ==
  data: x output; t input; y output; Tdur input; P0x input; P0z input; P1x input; P1z input; P2x input; P2z input; P3x input; P3z input
function [x, y] = bezTrajV2(t, Tdur, P0x,P0z,P1x,P1z,P2x,P2z,P3x,P3z)
t_swing = Tdur/4;
t_support = Tdur*3/4;

P0 = [P0x, P0z];
P1 = [P1x, P1z];
P2 = [P2x, P2z];
P3 = [P3x, P3z];
if t<=t_swing
    Sw = P0*((1-(t/t_swing))^3) + 3*P1*(t/t_swing)*((1-(t/t_swing))^2) + 3*P2*((t/t_swing)^2)*(1-(t/t_swing)) + P3*((t/t_swing)^3);
    
    x = -1*Sw(1);
    y = Sw(2);
else
    x = -1*(P3(1)+(P0(1)-P3(1))/t_support*(t-t_swing));
    y = -0.003*sin((x-P0(1))*pi/(P3(1)-P0(1)))+P0(2);
end
end

== matlab function gait_testing/Gait Selector/Turn Left Gait - Bezier Curves/Sin-Movement/MATLAB Function1 ==
  data: x input; theta1 output; y input; L1 input; L2 input; theta2 output
function [theta1, theta2] = ang(x,y,L1,L2)
theta2 = acos((x.^2+y.^2-L1.^2-L2.^2) / (2*L1*L2));
beta = asin((L2*sin(theta2))./((x.^2+y.^2).^0.5));
theta1 = asin(x./((x.^2+y.^2).^0.5)) + beta;
end

== matlab function gait_testing/Gait Selector/Turn Right Gait - Bezier Curves/Plane Movement/MATLAB Function1 ==
  data: x input; theta1 output; y input; L1 input; L2 input; theta2 output
function [theta1, theta2] = ang(x,y,L1,L2)
theta2 = acos((x.^2+y.^2-L1.^2-L2.^2) / (2*L1*L2));
beta = asin((L2*sin(theta2))./((x.^2+y.^2).^0.5));
theta1 = asin(x./((x.^2+y.^2).^0.5)) + beta;
end

== matlab function gait_testing/Gait Selector/Turn Right Gait - Bezier Curves/Plane Movement/MATLAB Function2 ==
  data: x output; t input; Tdur input; y output; P0x input; P0z input; P1x input; P1z input; P2x input; P2z input; P3x input; P3z input
function [x, y] = bez_plane_TrajV2(t,Tdur,P0x,P0z,P1x,P1z,P2x,P2z,P3x,P3z)
t_swing = Tdur/4;
t_support = Tdur*3/4;

P0 = [P0x, P0z];
P1 = [P1x, P1z];
P2 = [P2x, P2z];
P3 = [P3x, P3z];
if t<=t_swing
    Sw = P0*((1-(t/t_swing))^3) + 3*P1*(t/t_swing)*((1-(t/t_swing))^2) + 3*P2*((t/t_swing)^2)*(1-(t/t_swing)) + P3*((t/t_swing)^3);
    
    x = -1*Sw(1);
    y = Sw(2);
else
    x = -1*(P3(1)+(P0(1)-P3(1))/t_support*(t-t_swing));
    y = P0(2);
end
end

== matlab function gait_testing/Gait Selector/Turn Right Gait - Bezier Curves/Plane Movement1/MATLAB Function2 ==
  data: x output; t input; Tdur input; y output; P0x input; P0z input; P1x input; P1z input; P2x input; P2z input; P3x input; P3z input
function [x, y] = bez_plane_TrajV2(t,Tdur,P0x,P0z,P1x,P1z,P2x,P2z,P3x,P3z)
t_swing = Tdur/4;
t_support = Tdur*3/4;

P0 = [P0x, P0z];
P1 = [P1x, P1z];
P2 = [P2x, P2z];
P3 = [P3x, P3z];
if t<=t_swing
    Sw = P0*((1-(t/t_swing))^3) + 3*P1*(t/t_swing)*((1-(t/t_swing))^2) + 3*P2*((t/t_swing)^2)*(1-(t/t_swing)) + P3*((t/t_swing)^3);
    
    x = 1*Sw(1);
    y = Sw(2);
else
    x = 1*(P3(1)+(P0(1)-P3(1))/t_support*(t-t_swing));
    y = P0(2);
end
end

== matlab function gait_testing/Gait Selector/Turn Right Gait - Bezier Curves/Plane Movement2/MATLAB Function2 ==
  data: x output; t input; Tdur input; y output; P0x input; P0z input; P1x input; P1z input; P2x input; P2z input; P3x input; P3z input
function [x, y] = bez_plane_TrajV2(t,Tdur,P0x,P0z,P1x,P1z,P2x,P2z,P3x,P3z)
t_swing = Tdur/4;
t_support = Tdur*3/4;

P0 = [P0x, P0z];
P1 = [P1x, P1z];
P2 = [P2x, P2z];
P3 = [P3x, P3z];
if t<=t_swing
    Sw = P0*((1-(t/t_swing))^3) + 3*P1*(t/t_swing)*((1-(t/t_swing))^2) + 3*P2*((t/t_swing)^2)*(1-(t/t_swing)) + P3*((t/t_swing)^3);
    
    x = -1*Sw(1);
    y = Sw(2);
else
    x = -1*(P3(1)+(P0(1)-P3(1))/t_support*(t-t_swing));
    y = P0(2);
end
end

== matlab function gait_testing/Gait Selector/Turn Right Gait - Bezier Curves/Plane Movement3/MATLAB Function2 ==
  data: x output; t input; Tdur input; y output; P0x input; P0z input; P1x input; P1z input; P2x input; P2z input; P3x input; P3z input
function [x, y] = bez_plane_TrajV2(t,Tdur,P0x,P0z,P1x,P1z,P2x,P2z,P3x,P3z)
t_swing = Tdur/4;
t_support = Tdur*3/4;

P0 = [P0x, P0z];
P1 = [P1x, P1z];
P2 = [P2x, P2z];
P3 = [P3x, P3z];
if t<=t_swing
    Sw = P0*((1-(t/t_swing))^3) + 3*P1*(t/t_swing)*((1-(t/t_swing))^2) + 3*P2*((t/t_swing)^2)*(1-(t/t_swing)) + P3*((t/t_swing)^3);
    
    x = 1*Sw(1);
    y = Sw(2);
else
    x = 1*(P3(1)+(P0(1)-P3(1))/t_support*(t-t_swing));
    y = P0(2);
end
end
